simulink model "project12020a"  (R2021b)
settings: Solver=ode2  StartTime=0.0  StopTime=765  FixedStep=1  MaxStep=0.2  MinStep=1e-20  RelTol=1e-3
values from neighbouring files (symbols this model uses):
  A_F = 1.93    [init.m]
  C_0 = 0.015    [init.m]
  C_D = 0.35    [init.m]
  E_ess_max = E_batt_kW * 1000 * 3600    (= 7200000)    [init.m]
  eta_ess = 0.8    [init.m]
  g = 9.81    [init.m]
  G_diff = 0.268    [init.m]
  G_elec = 1    [init.m]
  grams_per_hr_to_gal_per_s = 9.778e-8    (= 9.778e-08)    [init.m]
  M_veh = M_glider + M_passengers + M_batt    (= 1976)    [init.m]
  mi_per_hr_to_m_per_s = 0.44704    [init.m]
  r_wheel = 0.2794    [init.m]
  rho = 1.225    [init.m]
  SOC_init = 0.5    [init.m]
undefined symbols (not defined in the file or in its folder): eng_map, hwfet, param
settings Model: Creator=wasynczu  LastModifiedBy=Arijeet
settings SolverCC: AlgebraicLoopSolver=TrustRegion
settings DebuggingCC: SFMachineParentedDataDiag=warning

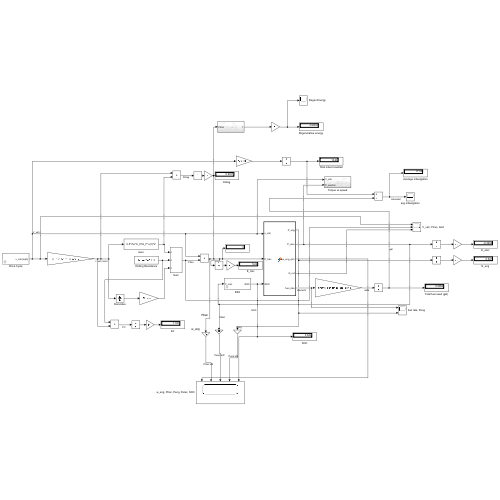
[thumbnail: Simulink's stored preview of the top-level diagram]
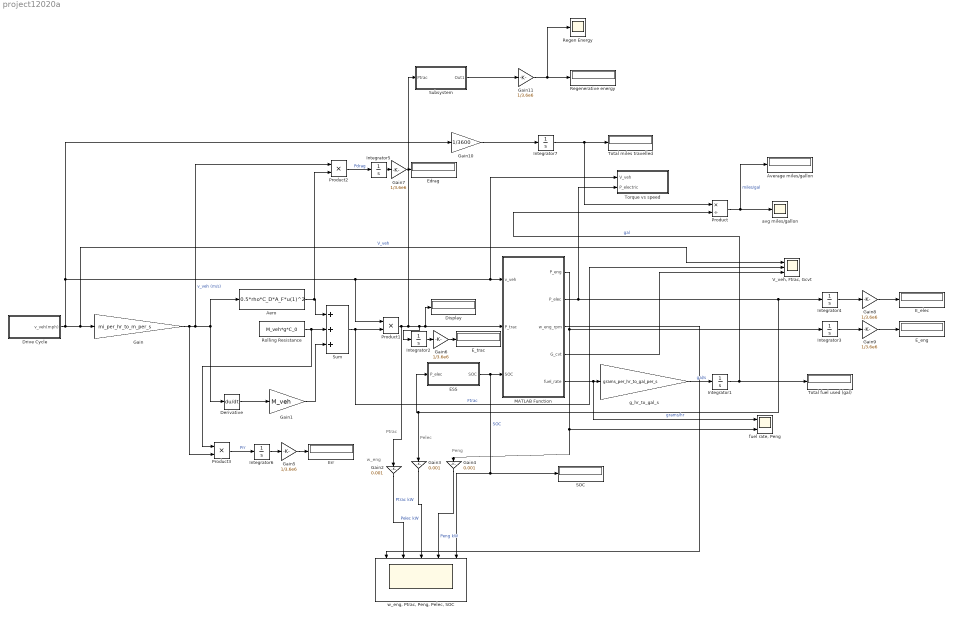
== system project12020a ==
  note: Ptrac
  note: Pelec
  note: Peng
  note: w_eng
  Aero : Fcn  Expr=0.5*rho*C_D*A_F*u(1)^2
  Average miles/gallon : Display
  Derivative : Derivative
  Display : Display
  Drive Cycle : Subsystem  mask{schedule=hwfet}
      mask prompts: schedule "drive schedule"
      mask init:
      | N=length(schedule(:,1));
  ESS : Subsystem  mask{E_max=E_ess_max, eta_ess=eta_ess}
      mask prompts: E_max "Maximum energy, J"; eta_ess "round-trip efficiency"
  E_elec : Display
  E_eng : Display
  E_trac : Display
  Edrag : Display
  Err : Display
  Gain : Gain  Gain=mi_per_hr_to_m_per_s
  Gain1 : Gain  Gain=M_veh
  Gain10 : Gain  Gain=1/3600
  Gain{5..9,11} (6 alike) : Gain  Gain=1/3.6e6
  Gain2 : Gain  Gain=0.001
  Gain3 : Gain  Gain=0.001
  Gain4 : Gain  Gain=0.001
  Integrator{1..7} (7 alike) : Integrator
  MATLAB Function : MATLAB Function  TreatAsAtomicUnit=on
  Product : Product  Inputs=*/
  Product1 : Product
  Product2 : Product
  Product3 : Product
  Regen Energy : Scope
  "Regenerative energy " : Display
  Rolling Resistance : Constant  Value=M_veh*g*C_0
  SOC : Display
  Subsystem : Subsystem
  Sum : Sum  Inputs=+++
  Torque vs speed : Subsystem
  Total fuel used (gal) : Display
  Total miles travelled : Display
  "V_veh, Ftrac, Gcvt" : Scope  NumInputPorts=3
  avg miles/gallon : Scope
  "fuel rate, Peng" : Scope  NumInputPorts=2
  g_hr_to_gal_s : Gain  Gain=grams_per_hr_to_gal_per_s
  "w_eng, Ptrac, Peng, Pelec, SOC" : Scope  NumInputPorts=5
  wires:
  Drive Cycle/1(v_veh(mph)) -> Gain10/1, Product1/1, Torque vs speed/1(V_veh), MATLAB Function/1(v_veh), "V_veh, Ftrac, Gcvt"/1, Gain/1  "V_veh"
  Derivative/1 -> Gain1/1
  Gain/1 -> Product3/2, Product2/1, Derivative/1, Aero/1  "v_veh (m/s)"
  Rolling Resistance/1 -> Product3/1, Sum/2
  Aero/1 -> Product2/2, Sum/1
  Gain1/1 -> Sum/3
  Sum/1 -> "V_veh, Ftrac, Gcvt"/2, Product1/2  "Ftrac"
  Product1/1 -> Subsystem/1(Ptrac), Integrator2/1, Display/1, MATLAB Function/2(P_trac), Gain2/1
  MATLAB Function/5(fuel_rate) -> "fuel rate, Peng"/1, g_hr_to_gal_s/1  "grams/hr"
  g_hr_to_gal_s/1 -> Integrator1/1  "gal/s"
  Integrator1/1 -> Total fuel used (gal)/1, Product/2  "gal"
  Product/1 -> Average miles/gallon/1, avg miles/gallon/1  "miles/gal"
  ESS/1(SOC) -> MATLAB Function/3(SOC), SOC/1, "w_eng, Ptrac, Peng, Pelec, SOC"/5  "SOC"
  MATLAB Function/3(w_eng_rpm) -> "w_eng, Ptrac, Peng, Pelec, SOC"/1
  Gain2/1 -> "w_eng, Ptrac, Peng, Pelec, SOC"/2  "Ptrac kW"
  Gain3/1 -> "w_eng, Ptrac, Peng, Pelec, SOC"/3  "Pelec kW"
  Gain4/1 -> "w_eng, Ptrac, Peng, Pelec, SOC"/4  "Peng kW"
  MATLAB Function/1(P_eng) -> Integrator3/1, Gain4/1, "fuel rate, Peng"/2
  MATLAB Function/4(G_cvt) -> "V_veh, Ftrac, Gcvt"/3
  MATLAB Function/2(P_elec) -> Torque vs speed/2(P_electric), Integrator4/1, ESS/1(P_elec), Gain3/1
  Product2/1 -> Integrator5/1  "Pdrag"
  Integrator6/1 -> Gain5/1
  Product3/1 -> Integrator6/1  "Prr"
  Gain5/1 -> Err/1
  Integrator2/1 -> Gain6/1
  Gain6/1 -> E_trac/1
  Integrator5/1 -> Gain7/1
  Gain7/1 -> Edrag/1
  Integrator4/1 -> Gain8/1
  Gain8/1 -> E_elec/1
  Integrator3/1 -> Gain9/1
  Gain9/1 -> E_eng/1
  Gain10/1 -> Integrator7/1
  Integrator7/1 -> Product/1, Total miles travelled/1
  Subsystem/1(Out1) -> Gain11/1
  Gain11/1 -> Regen Energy/1, "Regenerative energy "/1

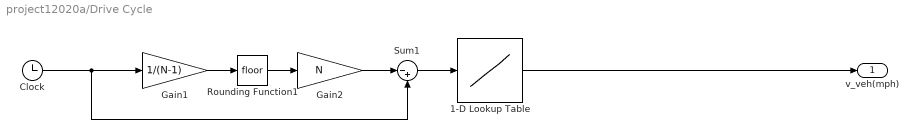
== system project12020a/Drive Cycle ==
  1-D Lookup Table : Lookup_n-D  NumberOfTableDimensions=1  BreakpointsForDimension1=schedule(:,1)  Table=schedule(:,2)  InterpMethod=Cubic spline  InternalRulePriority=Speed  RndMeth=Simplest  InputSameDT=on
  Clock : Clock
  Gain1 : Gain  Gain=1/(N-1)
  Gain2 : Gain  Gain=N
  Rounding Function1 : Rounding
  Sum1 : Sum  Inputs=|-+
  v_veh(mph) : Outport  VectorParamsAs1DForOutWhenUnconnected=off
  wires:
  Clock/1 -> Gain1/1, Sum1/2
  Sum1/1 -> 1-D Lookup Table/1
  Gain2/1 -> Sum1/1
  Rounding Function1/1 -> Gain2/1
  Gain1/1 -> Rounding Function1/1
  1-D Lookup Table/1 -> v_veh(mph)/1

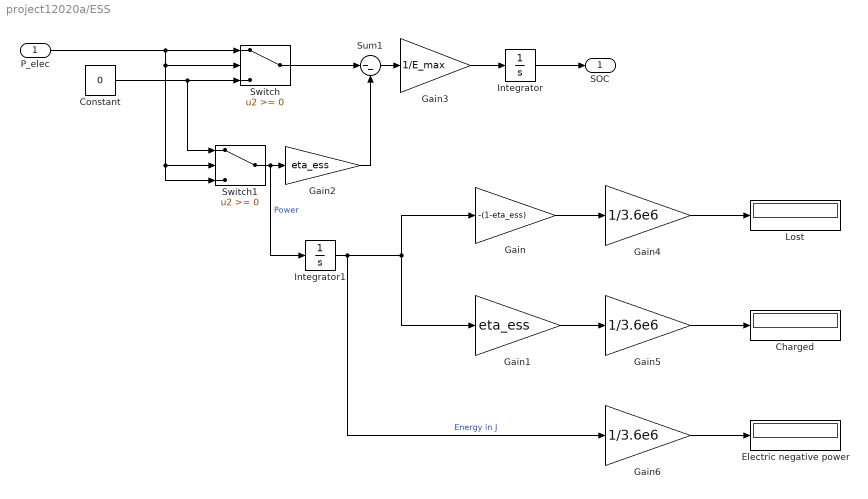
== system project12020a/ESS ==
  P_elec : Inport
  Charged : Display
  Constant : Constant  Value=0
  Electric negative power : Display
  Gain : Gain  Gain=-(1-eta_ess)
  Gain1 : Gain  Gain=eta_ess
  Gain2 : Gain  Gain=eta_ess
  Gain3 : Gain  Gain=1/E_max  OutDataTypeStr=fixdt('double', 'DataTypeOverride', 'Off')
  Gain4 : Gain  Gain=1/3.6e6
  Gain5 : Gain  Gain=1/3.6e6
  Gain6 : Gain  Gain=1/3.6e6
  Integrator : Integrator  InitialCondition=SOC_init  LimitOutput=on  UpperSaturationLimit=1  LowerSaturationLimit=0
  Integrator1 : Integrator
  Lost : Display
  Sum1 : Sum  Inputs=|--
  Switch : Switch  OutDataTypeStr=double
  Switch1 : Switch  OutDataTypeStr=double
  SOC : Outport  VectorParamsAs1DForOutWhenUnconnected=off
  wires:
  P_elec/1 -> Switch1/2, Switch1/3, Switch/2, Switch/1
  Gain3/1 -> Integrator/1
  Gain2/1 -> Sum1/2
  Switch1/1 -> Integrator1/1, Gain2/1  "Power"
  Sum1/1 -> Gain3/1
  Switch/1 -> Sum1/1
  Constant/1 -> Switch1/1, Switch/3
  Integrator/1 -> SOC/1
  Integrator1/1 -> Gain6/1, Gain/1, Gain1/1  "Energy in J"
  Gain/1 -> Gain4/1
  Gain1/1 -> Gain5/1
  Gain4/1 -> Lost/1
  Gain6/1 -> Electric negative power/1
  Gain5/1 -> Charged/1

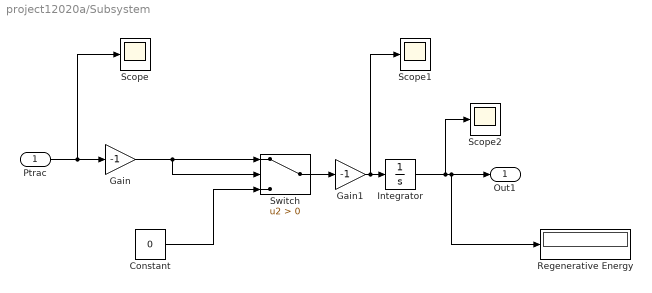
== system project12020a/Subsystem ==
  Ptrac : Inport
  Constant : Constant  Value=0
  Gain : Gain  Gain=-1
  Gain1 : Gain  Gain=-1
  Integrator : Integrator
  Regenerative Energy : Display
  Scope : Scope
  Scope1 : Scope
  Scope2 : Scope
  Switch : Switch  Criteria=u2 > Threshold
  Out1 : Outport
  wires:
  Ptrac/1 -> Scope/1, Gain/1
  Gain/1 -> Switch/2, Switch/1
  Constant/1 -> Switch/3
  Switch/1 -> Gain1/1
  Gain1/1 -> Scope1/1, Integrator/1
  Integrator/1 -> Scope2/1, Regenerative Energy/1, Out1/1

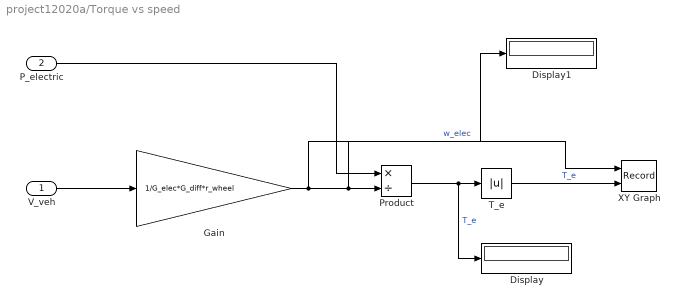
== system project12020a/Torque vs speed ==
  V_veh : Inport
  P_electric : Inport  Port=2
  Display : Display
  Display1 : Display
  Gain : Gain  Gain=1/G_elec*G_diff*r_wheel
  Product : Product  Inputs=*/
  T_e : Abs
  XY Graph : Record  FileSettingsInternal="{\"entries\":[{\"content\":{\"excelSettings\":{\"content\":{},\"type\":\"Streamout.ExcelSettings\"}},\"type\":\"Streamout.FileSettingStorage\",\"uuid\":\"9371f16c-9042-43f9-9f3b-7871b295fad2\"}],\"packageUris\":[\"http://schema.mathworks.com/mf0/streamout_blocks/R2020a\"],\"version\":\"1.0\"}"  Layout=[1 1]  SignalsInternal="{\"entries\":[{\"content\":{\"signals\":[{\"content\":{\"blockPath\":[\"project12020a/Torque vs speed/XY Graph\"],\"channel\":[],\"dimensions\":[1],\"domain\":\"project12020a/Torque vs speed/XY Graph\",\"lineColor\":\"#a2142f\",\"plots\":[1],\"port\":1,\"sid\":[\"\"],\"signalID\":864,\"signalName\":\"w_elec\"},\"type\":\"RecordBlkView.Signal\",\"uuid\":\"17ac89e1-f93b-4719-ba3f-bdfb878589d7\"},{\"content\":{\"blockPath\":[\"project12020a/Torque vs speed/XY Graph\"],\"channel\":[],\"dimensions\":[1],\"domain\":\"project12020a/Torque vs speed/XY Graph\",\"lineColor\":\"#139fff\",\"plots\":[1],\"port\":2,\"sid\":[\"\"],\"signalID\":868,\"signalName\":\"T_e\"},\"type\":\"RecordBlkView.Signal\",\"uuid\":\"23408d8e-4d50-4087-81d4-89ba304c0cdf\"}]},\"type\":\"RecordBlkView.InputSignals\",\"uuid\":\"905f18c6-c90c-47dc-9ced-aa38f2971279\"}],\"packageUris\":[\"http://schema.mathworks.com/mf0/streamout_blocks/R2020a\"],\"version\":\"1.0\"}"  VisualizationBindings="{\"xyplotplugin\":{\"info\":[{\"series\":[{\"bindingParametersList\":[{\"parameter\":\"X-Axis\",\"signalID\":864,\"signalName\":\"w_elec\"},{\"parameter\":\"Y-Axis\",\"signalID\":868,\"signalName\":\"T_e\"}],\"seriesID\":20207},{\"bindingParametersList\":[{\"parameter\":\"Y-Axis\",\"signalID\":864,\"signalName\":\"w_elec\"}],\"seriesID\":850}],\"subplotID\":1}]}}"  CompatibilityTag=XY
  wires:
  V_veh/1 -> Gain/1
  Gain/1 -> Display1/1, XY Graph/1, Product/2  "w_elec"
  P_electric/1 -> Product/1
  Product/1 -> Display/1, T_e/1  "T_e"
  T_e/1 -> XY Graph/2  "T_e"

== matlab function project12020a/MATLAB Function ==
  data: v_veh input; P_eng output; P_trac input; SOC input; P_elec output; w_eng_rpm output; G_cvt output; fuel_rate output; param parameter; eng_map parameter
function [P_eng, P_elec, w_eng_rpm, G_cvt, fuel_rate] = fcn(v_veh, P_trac, SOC, param, eng_map)
%#codegen
%inputs:
    % v_veh, m/s
    % P_trac, W
    % SOC
    % param, structure of parameters
    % eng_map

% outputs:
    %   P_gen, P_elec in W
    %   w_eng_rpm, rpm
    %   G_cvt (cvt ratio)
    %   Fuel rate, grams/hr

v_veh_min = param.v_veh_min;    % minimum vehicle speed for engine to stay engaged, in m/s
P_eng_min = param.P_eng_min;    % minimum engine power in W
P_eng_max = param.P_eng_max ;   % maximum engine power
G_cvt_min = param.G_cvt_min;    % minimum cvt  ratio
G_diff = param.G_diff;          % differential gear ratio
r_wheel = param.r_wheel;        % wheel radius in m

if (v_veh < v_veh_min)  % disengage clutch, idle engine, electric propulsion
   P_elec = P_trac;
   P_eng = 0;
   fuel_rate = 0; % g/hr;
   w_eng_rpm = 1000; % rpm
   G_cvt = G_cvt_min;
   return  
end

% if here, v_veh > v_veh_min
if(P_trac < P_eng_min)   % clutch engaged but engine idling
   P_elec = P_trac;
   fuel_rate = 0;
   P_eng = 0;
   w_eng_rpm =  1000; % rpm
   w_eng = w_eng_rpm * pi / 30; % rad/s
   % set G_cvt so engine speed is 1000 rpm
   G_cvt = v_veh/G_diff/w_eng/r_wheel;
   return     
end

if(P_trac > P_eng_max) % high-speed boost
   P_elec = P_trac - P_eng_max;
   P_eng = P_eng_max;
   bsfc = interp1(eng_map(:,2), eng_map(:,3), P_eng/1000, 'pchip', 'extrap');
   fuel_rate = bsfc*P_eng/1000; % grams/hr
   w_eng_rpm = interp1(eng_map(:,2), eng_map(:,1), P_eng/1000, 'pchip', 'extrap');
   w_eng = w_eng_rpm * pi / 30; % convert to rad/s
   G_cvt =  v_veh/r_wheel/G_diff/w_eng; % required CVT ratio
   return   
end

% if here, v_veh > v_veh_min and P_eng_min < P_trac < P_eng_max
% try to get SOC back to 0.5

P_elec = 20000*(SOC - 0.5); 
if(P_elec > 4000)
    P_elec = 4000;
end
if(P_elec < -4000)
    P_elec = -4000;
end

P_eng = P_trac - P_elec;


if(P_eng < P_eng_min) 
   % clutch engaged, but no fuel
   P_eng = 0;
   P_elec = P_trac;
   fuel_rate = 0;
   w_eng_rpm = 1000;
   w_eng = w_eng_rpm * 2 * pi / 60; % in rad/s
   % set G_cvt so engine speed is 1000 rpm
   G_cvt = v_veh/G_diff/w_eng/r_wheel;
   return
end

if(P_eng > P_eng_max)
    P_eng = P_eng_max;
    P_elec = P_trac - P_eng_max;
end

bsfc = interp1(eng_map(:,2), eng_map(:,3), P_eng/1000, 'pchip', 'extrap');
fuel_rate = bsfc*P_eng/1000; % grams/hr

w_eng_rpm = interp1(eng_map(:,2), eng_map(:,1), P_eng/1000, 'pchip', 'extrap');
if(w_eng_rpm < 1000)
    w_eng_rpm = 1000;
end
w_eng = w_eng_rpm * pi / 30;  % convert to rad/s
G_cvt =  v_veh/r_wheel/G_diff/w_eng;

if (G_cvt < G_cvt_min) % set G_cvt = G_cvt_min, recalculate w_eng, P_eng, and P_elec
   G_cvt = G_cvt_min;
   w_eng = v_veh/G_diff/r_wheel/G_cvt;
   w_eng_rpm = w_eng*30/pi;  % in rpm
   P_eng = 1000*interp1(eng_map(:,1), eng_map(:,2), w_eng, 'pchip', 'extrap'); % in W
   if(P_eng < 0)
       P_eng = 0;
   end
   P_elec = P_trac - P_eng;
   bsfc = interp1(eng_map(:,1), eng_map(:,3), w_eng, 'pchip', 'extrap');
   fuel_rate = bsfc*P_eng/1000; % grams/hr
 end
